simulink model "lifxudp_SLX"  (R2016b)
settings: Solver=ode5  StartTime=0.0  StopTime=inf  FixedStep=0.001  RelTol=1e-3  EnableMultiTasking=on
undefined symbols (not defined in the file or in its folder): Standard_Devices, UDP_Protocol
libraries: sldrtlib x1
settings Model: SimulationMode=external  Creator=julianleland  LastModifiedBy=julianleland
settings OptimizationCC: LifeSpan=inf
settings DebuggingCC: SFUnexpectedBacktrackingDiag=warning  SFNoUnconditionalDefaultTransitionDiag=warning  SFExecutionAtInitializationDiag=none
settings HardwareCC: ProdBitPerLong=64  ProdHWDeviceType=Intel->x86-64 (Mac OS X)  TargetBitPerLong=64  TargetBitPerPointer=64  TargetIntDivRoundTo=Zero  TargetEndianess=LittleEndian  TargetWordSize=64  TargetHWDeviceType=Intel->x86-64
settings RTWCC: SystemTargetFile=sldrt.tlc  TemplateMakefile=sldrt.tmf  Description=Simulink Desktop Real-Time  RTWCompilerOptimization=on
settings CodeAppCC: MaxIdLength=95
settings SimulinkDesktopRealTimeCC: TargetPreCompLibLocation=/Applications/MATLAB_R2016b.app/toolbox/sldrt/lib/maci64  TargetLangStandard=C89/C90 (ANSI)  SupportVariableSizeSignals=off
settings ConfigComp: CovMetricSettings=dw  CovHtmlReporting=on  CovSaveCumulativeToWorkspaceVar=on  CovSaveSingleToWorkspaceVar=on  CovExternalEMLEnable=off

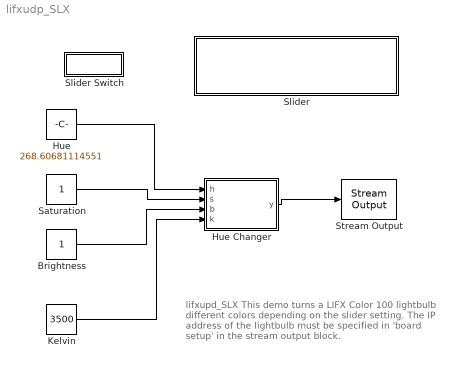
== system lifxudp_SLX ==
  note: lifxupd_SLX
      |
      | This demo turns a LIFX Color 100 lightbulb different colors depending on the slider setting.
      | The IP address of the lightbulb must be specified in 'board setup' in the stream output block.
  "Brightness " : Constant  OutMax=[1]  OutDataTypeStr=double
  "Hue " : Constant  Value=268.60681114551  OutMin=[0]  OutMax=[360]  OutDataTypeStr=double
  Hue Changer : MATLAB Function  TreatAsAtomicUnit=on
  Kelvin : Constant  Value=3500  OutMin=[2500]  OutMax=[9000]  OutDataTypeStr=double
  Saturation : Constant  OutDataTypeStr=double
  Slider : Subsystem  DialogController=hmiCreateDDGDialog  IsWebBlock=on  mask(MWDashboardBlock){webBlockId=9f94ac96-0546-4ef9-a244-4590f8043070, webBlockType=slider, ShowInLibBrowser=on, ShowInitialText=on, HMISrcModelName=lifxudp_SLX}
      mask prompts: webBlockId "WebBlock Id"; webBlockType "WebBlock Type"; HMISrcModelName "Source Model"
      mask help: SimulinkHMI:dialogs:SliderDialogDesc
      mask Help: helpview([docroot '/mapfiles/simulink.map'], 'hmi_slider')
      mask Display:
      | if strcmp(get_param(bdroot(gcb),'BlockDiagramType'), 'library')
      |     image([(matlabroot) '/toolbox/simulink/hmi/icons/Slider.png']);
      | end
  Slider Switch : Subsystem  DialogController=hmiCreateDDGDialog  IsWebBlock=on  mask(MWDashboardBlock){webBlockId=6db1f250-b783-43d1-b21c-aef7d5068c72, webBlockType=sliderswitch, ShowInLibBrowser=on, ShowInitialText=on, HMISrcModelName=lifxudp_SLX}
      mask prompts: webBlockId "WebBlock Id"; webBlockType "WebBlock Type"; HMISrcModelName "Source Model"
      mask help: SimulinkHMI:dialogs:SwitchDialogDesc
      mask Help: helpview([docroot '/mapfiles/simulink.map'], 'hmi_slider_switch')
      mask Display:
      | if strcmp(get_param(bdroot(gcb),'BlockDiagramType'), 'library')
      |     image([(matlabroot) '/toolbox/simulink/hmi/icons/SliderSwitch.png']);
      | end
  Stream Output : sldrtlib/Stream Output  SampleTime=.1  MaxMissedTicks=10  ShowMissedTicks=off  YieldWhenWaiting=off  DrvName=Standard_Devices/UDP_Protocol  DrvAddress=54359  DrvOptions=[174338150 56700]  PortSizes=49  FormatString=repmat('%c',1,49)  ShowReady=off  ShowError=off  InitialValue=[]  FinalValue=[]
      settings: AttributesFormatString=Standard Devices\nUDP Protocol [D457h]
  wires:
  Hue Changer/1(y) -> Stream Output/1
  "Hue "/1 -> Hue Changer/1(h)
  Saturation/1 -> Hue Changer/2(s)
  "Brightness "/1 -> Hue Changer/3(b)
  Kelvin/1 -> Hue Changer/4(k)

== system lifxudp_SLX/Slider ==

== system lifxudp_SLX/Slider Switch ==

== matlab function lifxudp_SLX/Hue Changer ==
  data: h input; y output size=[1,49]; s input; b input; k input
function y = fcn(h,s,b,k)
%#codegen
%%
dec_code = [49;0;0;52;0;0;0;0;0;0;0;0;0;0;0;0;0;0;0;0;0;0;0;0;0;0;0;0;0;0;0;0;102;0;0;0;0;85;85;255;255;255;255;191;218;0;0;0;0];
%%
%%HUE 
hue = h/360 * 65535; %hue conversion formula, from degrees scale to LIFX scale
hue = floor(hue);
hue_hex = dec2hex(hue);

if (length(hue_hex) == 1)
    hue_arr = ['0',hue_hex(1)];
    hue_arr = ['00',hue_arr(1:2)];

elseif (length(hue_hex) ==2)
    hue_arr = ['00',hue_hex(1:2)];  
    
elseif (length(hue_hex) == 3)
    hue_arr = ['0', hue_hex(1), hue_hex(2), hue_hex(3)];
    hue_arr = [hue_arr(1:2),hue_arr(3:4)];
    
else
    hue_arr = [hue_hex(1:2), hue_hex(3:4)];
        
end

hue_out = hex2dec(hue_arr(1:2));
hue_out2 = hex2dec(hue_arr(3:4));

dec_code(38) = hue_out2;
dec_code(39) = hue_out;

%%
%SATURATION
sat = s * 65535; %saturation conversion formula, from 0-1 to LIFX scale
sat = floor(sat);
sat_hex = dec2hex(sat);

if (length(sat_hex) == 1)
    sat_arr = ['0',sat_hex(1)];
    sat_arr = ['00',sat_arr(1:2)];

elseif (length(sat_hex) ==2)
    sat_arr = ['00',sat_hex(1:2)];  
    
elseif (length(sat_hex) == 3)
    sat_arr = ['0', sat_hex(1), sat_hex(2), sat_hex(3)];
    sat_arr = [sat_arr(1:2),sat_arr(3:4)];
    
else
    sat_arr = [sat_hex(1:2), sat_hex(3:4)];
        
end

sat_out = hex2dec(sat_arr(1:2));
sat_out2 = hex2dec(sat_arr(3:4));

dec_code(40) = sat_out2;
dec_code(41) = sat_out;

%%

%BRIGHTNESS
bright = b * 65535; %brightness conversion formula, from 0-1 to LIFX scale
bright = floor(bright);
bright_hex = dec2hex(bright);

if (length(bright_hex) == 1)
    bright_arr = ['0',bright_hex(1)];
    bright_arr = ['00',bright_arr(1:2)];

elseif (length(bright_hex) ==2)
    bright_arr = ['00',bright_hex(1:2)];  
    
elseif (length(bright_hex) == 3)
    bright_arr = ['0', bright_hex(1), bright_hex(2), bright_hex(3)];
    bright_arr = [bright_arr(1:2),bright_arr(3:4)];
    
else
    bright_arr = [bright_hex(1:2), bright_hex(3:4)];
end

bright_out = hex2dec(bright_arr(1:2));
bright_out2 = hex2dec(bright_arr(3:4));

dec_code(42) = bright_out2;
dec_code(43) = bright_out;

%%
%KELVIN
kelvin = k; %Kelvin conversion formula, from 0-1 to LIFX scale
kelvin = floor(kelvin);
kelvin_hex = dec2hex(kelvin);

if (length(kelvin_hex) == 1)
    kelvin_arr = ['0',kelvin_hex(1)];
    kelvin_arr = ['00',kelvin_arr(1:2)];

elseif (length(kelvin_hex) ==2)
    kelvin_arr = ['00',kelvin_hex(1:2)];  
    
elseif (length(kelvin_hex) == 3)
    kelvin_arr = ['0', kelvin_hex(1), kelvin_hex(2), kelvin_hex(3)];
    kelvin_arr = [kelvin_arr(1:2), kelvin_arr(3:4)];
    
else
    kelvin_arr = [kelvin_hex(1:2), kelvin_hex(3:4)];
end

kelvin_out = hex2dec(kelvin_arr(1:2));
kelvin_out2 = hex2dec(kelvin_arr(3:4));

dec_code(44) = kelvin_out2;
dec_code(45) = kelvin_out;

%%
%y_temp = char_out;
%y = y_temp(1:2);

y = uint8(dec_code');
